simulink model "test_data_acquisition"  (R2014a)
settings: Solver=ode45  StartTime=0.0  StopTime=5  RelTol=1e-3
libraries: TEsim_utils x4
settings Model: Creator=rnc4  LastModifiedBy=rnc4

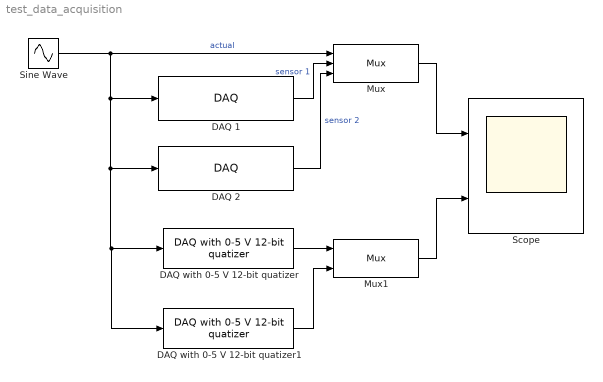
== system test_data_acquisition ==
  DAQ 1 : TEsim_utils/DAQ  frame_dur_sec=0.1  timeslot_offset_ms=51
  DAQ 2 : TEsim_utils/DAQ  frame_dur_sec=0.1  timeslot_offset_ms=10
  DAQ with 0-5 V 12-bit quatizer : TEsim_utils/DAQ with  0-5 V 12-bit quatizer  frame_dur_sec=0.1  timeslot_offset_ms=10  NumberOfConverterBits=8  Vmin=0  Vmax=5  Gain=0.5
  DAQ with 0-5 V 12-bit quatizer1 : TEsim_utils/DAQ with  0-5 V 12-bit quatizer  frame_dur_sec=0.1  timeslot_offset_ms=10  NumberOfConverterBits=8  Vmin=0  Vmax=5  Gain=0.1
  Mux : Mux  Inputs=3
      settings: DisplayOption=signals
  Mux1 : Mux  Inputs=2
      settings: DisplayOption=signals
  Scope : Scope  NumInputPorts=2
      settings: ShowLegends=on  TimeRange=5  YMin=0~0  YMax=5~4500
  Sine Wave : Sin  Amplitude=2.5  Bias=2.5  Frequency=0.5*pi  SampleTime=1/1000
  wires:
  Sine Wave/1 -> DAQ with 0-5 V 12-bit quatizer1/1, DAQ with 0-5 V 12-bit quatizer/1, DAQ 2/1, DAQ 1/1, Mux/1  "actual"
  DAQ 1/1 -> Mux/2  "sensor 1"
  DAQ 2/1 -> Mux/3  "sensor 2"
  Mux/1 -> Scope/1
  DAQ with 0-5 V 12-bit quatizer/1 -> Mux1/1
  DAQ with 0-5 V 12-bit quatizer1/1 -> Mux1/2
  Mux1/1 -> Scope/2
